simulink model "ProvaSCADA"  (R2024b)
settings: Solver=FixedStepAuto  StartTime=0.0  StopTime=Tsim  FixedStep=dT  RelTol=1e-3
values from neighbouring files (symbols this model uses):
  b = t + 2*s    (= 3.6)    [ParametriSegheria.m]    (also in ParametriSegheriaDinamica.m)
  h_index = [70, 80, 90, 100]    [ParametriSegheria.m]    (also in ParametriSegheriaDinamica.m)
  J1 = 8*1e6    (= 8000000)    [ParametriSegheriaDinamica.m]
  J2 = 0.9*1e6    (= 900000)    [ParametriSegheriaDinamica.m]
  kc = [0 35 40 50 55 90]    [ParametriSegheria.m]    (also in ParametriSegheriaDinamica.m = [0, 25, 30, 35, 50, 70])
  Kt = 2    [ParametriSegheria.m]    (also in ParametriSegheriaDinamica.m = 10000)
  Kt2 = 5    [ParametriSegheria.m]    (also in ParametriSegheriaDinamica.m = 4500)
  l_index = [20, 30, 40, 50]    [ParametriSegheria.m]    (also in ParametriSegheriaDinamica.m)
  Lt = 4    [ParametriSegheria.m]    (also in ParametriSegheriaDinamica.m)
  Mag_D = [0 430 320 260 230 540 430 320 260 230 540 430 320 260 230 540 430 320 260 230 540 430 320 260 230 540 430 320 260 230 540]    [ParametriSegheria.m]    (also in ParametriSegheriaDinamica.m = [0 randi([220 500], 1, 150)])
  Mag_legno = [0 1 5 2 4 3 1 5 2 4 3 1 5 2 4 3 1 5 2 4 3 1 5 2 4 3 1 5 2 4 3]    [ParametriSegheria.m]    (also in ParametriSegheriaDinamica.m = [0 randi([1 5], 1, 150)])
  n_sottili = 4    [ParametriSegheria.m]    (also in ParametriSegheriaDinamica.m)
  omega_ref1 = 50    [ParametriSegheriaDinamica.m]
  omega_ref2 = 3000*(2*pi/60)    (= 314.159265359)    [ParametriSegheriaDinamica.m]
  Rc = 200    [ParametriSegheria.m]    (also in ParametriSegheriaDinamica.m)
  rho = [0, 450, 520, 590, 710, 780]*1e-9    [ParametriSegheriaDinamica.m]
  Rs = 800    [ParametriSegheria.m]    (also in ParametriSegheriaDinamica.m)
  SR = Rs/Rm    (= 5.33333333333)    [ParametriSegheria.m]    (also in ParametriSegheriaDinamica.m)
  SR2 = Rc/Rm2    (= 4)    [ParametriSegheria.m]    (also in ParametriSegheriaDinamica.m)
undefined symbols (not defined in the file or in its folder): thrsh
libraries: simulink x6, slpidlib x6
(part 2 of 2)

== matlab function ProvaSCADA/Subsystem1/MATLAB Function3 ==
  data: h_next output; l_next output; Magazzino output; h_idx input; l_idx input; target_matrice parameter; n_assi input; work output
function [h_next, l_next, Magazzino, work] = fcn(h_idx, l_idx, target_matrice, n_assi)

[n_rows, n_cols] = size(target_matrice);

h_next = zeros(1,length(h_idx));
l_next = zeros(1,length(l_idx));

persistent MagazzinoGlobale

for i = 1:length(n_assi)

    if isempty(MagazzinoGlobale)
        MagazzinoGlobale = zeros(n_rows, n_cols);
    end
    
    
    % Output iniziali
    h_next(i) = h_idx(i);
    l_next(i) = l_idx(i);
    
    
    MagazzinoGlobale(h_idx(i), l_idx(i)) = MagazzinoGlobale(h_idx(i), l_idx(i)) + n_assi(i);
    
    work = 1;
    
    if MagazzinoGlobale(h_idx(i), l_idx(i)) >= target_matrice(h_idx(i), l_idx(i))
    
        % Quanto manca a completare ogni cella
        deficit = target_matrice - MagazzinoGlobale;
        
        % Trova la cella con massimo deficit
        [max_val, linear_idx] = sort(deficit(:), 'descend');
        
        if (max_val(1) > 0)
            [h_next(i), l_next(i)] = ind2sub(size(deficit), linear_idx(i));
        else
            % Tutto completato (magazzino riempito): rimani sulla stessa
            % cella + ferma
            h_next(i) = h_idx(i);
            l_next(i) = l_idx(i);
            work = 0;
        end
    end
end

Magazzino = MagazzinoGlobale;
